simulink model "pressPedal"  (R2015b)
settings: Solver=VariableStepAuto  StartTime=0.0  StopTime=10.0  RelTol=1e-3
settings Model: Creator=Josef  LastModifiedBy=Josef

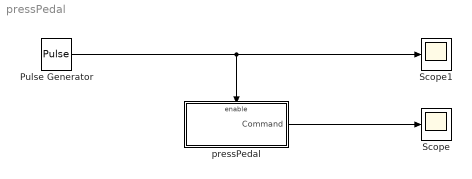
== system pressPedal ==
  Pulse Generator : DiscretePulseGenerator  PulseType=Time based  PulseWidth=30
  Scope : Scope
  Scope1 : Scope
  pressPedal : Subsystem
  wires:
  Pulse Generator/1 -> Scope1/1, pressPedal/Enable
  pressPedal/1(Command) -> Scope/1

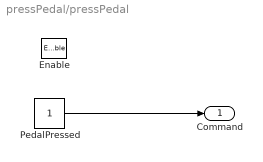
== system pressPedal/pressPedal ==
  Enable : EnablePort
  PedalPressed : Constant
  Command : Outport  OutputWhenDisabled=reset  InitialOutput=0
  wires:
  PedalPressed/1 -> Command/1
